simulink model "covering_1_newAxis"  (R2017b)
settings: Solver=VariableStepAuto  StartTime=0.0  StopTime=400  FixedStep=0.0000001  RelTol=1e-3
undefined symbols (not defined in the file): Cwy1, Cwy2, Cx, Jyy, k1_k, k2_k, k2_m, K_thruster, kc, L, lambda11, lambda55, m, Rmin, T_thruster, Vz
libraries: simulink x6, simulink_extras x1
settings Model: PauseTimes=70  NumberOfSteps=10  Creator=Eugene  LastModifiedBy=Eugene
settings DebuggingCC: ParameterOverflowMsg=warning
settings HardwareCC: ProdHWDeviceType=AMD->x86-64 (Windows64)

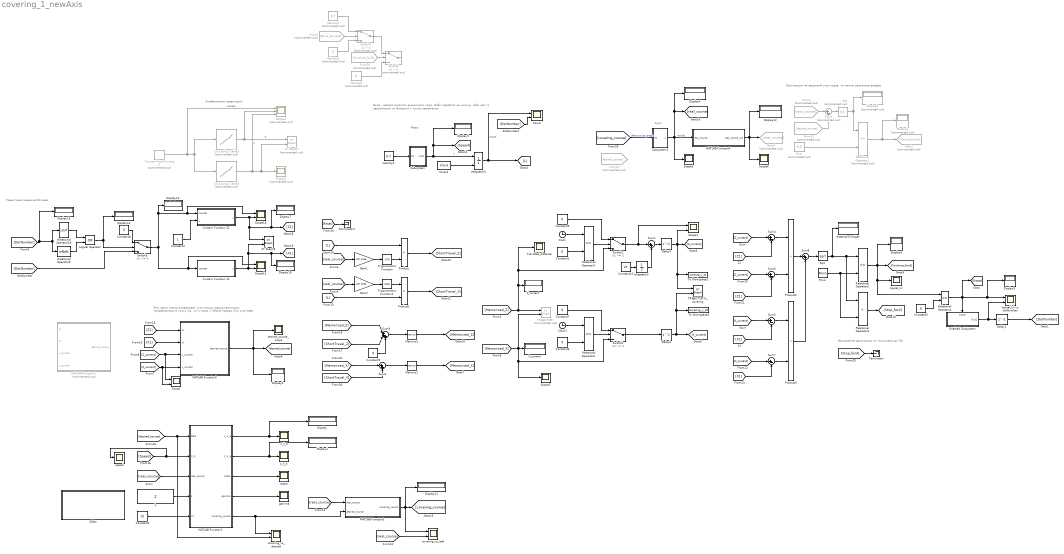
== system covering_1_newAxis ==
  note: Вход - всегда скорость экономного хода. Либо подаётся на контур, либо нет, в зависимости от близости к точке назначения
  note: Марш
  note: angle
  note: Курс
  note: Отображение траектории
  note: Вычисление расстояния от точки-цели до ПА
  note: Если вышли на заданный угол курса, то можно двигаться вперёд
  note: Траектория через switch-case
  note: Эта часть схемы определяет угол между радиус-вектором, направленным в точку (z1, x1) и осью z. Иначе говоря, это угол beta
  1-D Lookup Table2 : Lookup_n-D  Commented=on  NumberOfTableDimensions=1  BreakpointsForDimension1=[0:7]  BreakpointsForDimension1FirstPoint=0  BreakpointsForDimension1DataTypeStr=uint8  Table=[0,0,L,L,2*L,2*L,3*L, 3*L]  TableDataTypeStr=double  InterpMethod=Flat  ExtrapMethod=Cubic spline  RemoveProtectionInput=on  InternalRulePriority=Speed  OutDataTypeStr=double  RndMeth=Zero  InputSameDT=on
  1-D Lookup Table3 : Lookup_n-D  Commented=on  NumberOfTableDimensions=1  BreakpointsForDimension1=[0:7]  BreakpointsForDimension1DataTypeStr=int16  Table=[0,25,25,0,0,25,25,0]  TableDataTypeStr=double  InterpMethod=Flat  RemoveProtectionInput=on  InternalRulePriority=Speed  OutDataTypeStr=double  RndMeth=Zero  InputSameDT=on
  Abs : Abs  Commented=on
  Clock : Clock
  Clock1 : Clock
  Clock2 : simulink_extras/Flip Flops/Clock  period=0.05
  Constant{1,3,5..9} (7 alike) : Constant  Value=0
  Constant10 : Constant  Value=Vz
  Constant2 : Constant  Value=Vz
  Constant4 : Constant  Value=L
  Counter Free-Running2 : simulink/Sources/Counter Free-Running  Commented=on  NumBits=3  tsamp=1
  Custom Function X1 : MATLAB Function  TreatAsAtomicUnit=on
  Custom Function Z1 : MATLAB Function  TreatAsAtomicUnit=on
  Delay1 : Delay  DelayLength=1  SampleTime=0.05
  Delay3 : Delay  DelayLength=1  SampleTime=0.05
  Delay4 : Delay  DelayLength=1  SampleTime=0.05
  Display{,1..2,4..7,9..15} (14 alike) : Display
  Display3 : Display  Commented=on
  Display8 : Display  Commented=on
  Enabled Subsystem : Subsystem  TreatAsAtomicUnit=on
  Error : Constant  Commented=on  Value=0.5
  From11 : From  Commented=on  GotoTag=desired_course
  From2 : From  Commented=on  GotoTag=Move_forward
  From27 : From  Commented=on  GotoTag=desired_course
  From29 : From  Commented=on  GotoTag=Continue_fwrd
  From4 : From  Commented=on  GotoTag=real_course
  Gain1 : Gain  Gain=1/57.2958
  Gain2 : Gain  Gain=1/57.2958
  Goto2 : Goto  Commented=on  GotoTag=Move_forward
  Goto4 : Goto  Commented=on  GotoTag=real_course
  Integrator2 : Integrator
  Integrator3 : Integrator  ExternalReset=rising
  Logical Operator : Logic  Operator=OR  AllPortsSameDT=off  OutDataTypeStr=boolean
  MATLAB Function1 : MATLAB Function  TreatAsAtomicUnit=on
  MATLAB Function2 : MATLAB Function  Commented=on  TreatAsAtomicUnit=on
  MATLAB Function3 : MATLAB Function  TreatAsAtomicUnit=on
  MATLAB Function4 : MATLAB Function  TreatAsAtomicUnit=on
  MATLAB Function5 : MATLAB Function  TreatAsAtomicUnit=on
  Memory1 : Memory
  Memory2 : Memory
  Product{,1..3} (4 alike) : Product
  Relational Operator1 : RelationalOperator  Commented=on  Operator=<=  OutDataTypeStr=boolean  RndMeth=Simplest
  Relational Operator10 : RelationalOperator  Operator=isInf  OutDataTypeStr=boolean  RndMeth=Simplest
  Relational Operator2 : RelationalOperator  OutDataTypeStr=boolean  RndMeth=Simplest
  Relational Operator3 : RelationalOperator  Operator=<  OutDataTypeStr=boolean  RndMeth=Simplest
  Relational Operator4 : RelationalOperator  Operator===  OutDataTypeStr=boolean  RndMeth=Simplest
  Relational Operator5 : RelationalOperator  Operator===  OutDataTypeStr=boolean  RndMeth=Simplest
  Relational Operator6 : RelationalOperator  Operator===  OutDataTypeStr=boolean  RndMeth=Simplest
  Relational Operator9 : RelationalOperator  Operator=isNaN  OutDataTypeStr=boolean  RndMeth=Simplest
  Rmin : Constant  Value=Rmin
  Scope{,1,13..14} (4 alike) : Scope  NumInputPorts=2
  Scope2 : Scope
  Scope3 : Scope  Commented=on  NumInputPorts=3
  Scope4 : Scope  Commented=on
  Scope5 : Scope
  Scope6 : Scope
  Slider : Subsystem  DialogController=hmiCreateDDGDialog  IsWebBlock=on  mask(MWDashboardBlock){webBlockId=306e3f62-3226-42d7-8a36-5c4e99ff92fc, webBlockType=slider, ShowInLibBrowser=on, ShowInitialText=on, HMISrcModelName=covering_1_newAxis}
      mask prompts: webBlockId "WebBlock Id"; webBlockType "WebBlock Type"; HMISrcModelName "Source Model"
      mask help: SimulinkHMI:dialogs:SliderDialogDesc
      mask Help: helpview([docroot '/mapfiles/simulink.map'], 'hmi_slider')
      mask Display:
      | if strcmp(get_param(bdroot(gcb),'BlockDiagramType'), 'library')
      |     image([(matlabroot) '/toolbox/simulink/hmi/icons/Slider.png']);
      | end
  Sqrt : Sqrt  SaturateOnIntegerOverflow=on
  Subsystem : Subsystem
  Subsystem1 : Subsystem
  Sum1 : Sum  Inputs=|++
  Sum2 : Sum  Inputs=|++
  Sum3 : Sum  Commented=on  Inputs=|+-
  Sum{4..7} (4 alike) : Sum  Inputs=|+-
  Sum8 : Sum  Inputs=|++
  Sum9 : Sum  Inputs=|+++
  Switch2 : Switch  Threshold=1
  Switch3 : Switch  Threshold=1
  Switch4 : Switch  Commented=on  Criteria=u2 > Threshold
  Switch5 : Switch  Threshold=1
  Switch6 : Switch  Commented=on  Criteria=u2 > Threshold
  TRAJECTORY : simulink/Sinks/XY Graph  Commented=on  xmin=-1  xmax=10  ymin=-5  ymax=30  st=-1
  TRAJECTORY1_covering : simulink/Sinks/XY Graph  xmin=-1  xmax=10  ymin=-5  ymax=30  st=-1
  Terminator : Terminator
  Terminator1 : Terminator
  To Workspace2 : ToWorkspace  VariableName=covering_z_10  SampleTime=-1
  To Workspace3 : ToWorkspace  VariableName=covering_x_10  SampleTime=-1
  Travelled_distance : Scope
  Trigonometric Function : Trigonometry
  Trigonometric Function1 : Trigonometry  Operator=cos
  Velocity2 : Constant  Value=0.7
  Velocity4 : Constant  Commented=on  Value=0
  Velocity5 : Constant  Commented=on  Value=0.7
  Velocity6 : Constant  Commented=on  Value=0
  XY Graph1 : simulink/Sinks/XY Graph  Commented=on  xmin=-10  xmax=20  ymin=-10  ymax=30  st=-1
  XY Graph5 : simulink/Sinks/XY Graph  xmin=-1  xmax=10  ymin=-5  ymax=30  st=-1
  X_current : Display
  Z_current : Display
  alpha : Scope
  covering_vs_desired : Scope  NumInputPorts=2
  covering_vs_real : Scope  NumInputPorts=2
  desired_course_scope : Scope
  distanceToTarget : Display
  gamma : Scope
  k : Constant  Value=2
  logical_lvl : Scope
  logical_lvl vs dotNumber : Scope  NumInputPorts=2
  "speed " : Scope
  travel : Scope  NumInputPorts=2
  x_V_a : Scope
  z_V_a : Scope
  wires:
  1-D Lookup Table3/1 -> Scope4/1, XY Graph1/2, Scope3/3  "X"
  1-D Lookup Table2/1 -> XY Graph1/1, Scope3/2  "Z"
  Counter Free-Running2/1 -> Scope3/1, 1-D Lookup Table2/1, 1-D Lookup Table3/1  "counter"
  Subsystem/1(Out1) -> [Speed], Display5/1, Integrator3/1  "V"
  [covering_course] -> Subsystem1/1(In1)  "delta course_angle"
  Subsystem1/1(Out1) -> [real_course], Display4/1, Scope5/1, MATLAB Function4/1(real_course)
  Trigonometric Function/1 -> Product/2
  [real_course] -> Gain1/1
  [real_course] -> Gain2/1
  Trigonometric Function1/1 -> Product1/1
  Integrator3/1 -> [L], travel/1  "travel"
  From4/1 -> Sum3/1
  From11/1 -> Sum3/2
  Sum3/1 -> Abs/1
  Error/1 -> Relational Operator1/2
  Relational Operator1/1 -> Goto2/1, Display3/1
  [L] -> Product1/2
  [L] -> Product/1
  Gain1/1 -> Trigonometric Function/1
  Gain2/1 -> Trigonometric Function1/1
  [Z_current] -> Sum4/1
  [Z1] -> Sum4/2
  [X_current] -> Sum5/1
  [X1] -> Sum5/2
  [Z1] -> Sum6/2
  [Z_current] -> Sum6/1
  Sum4/1 -> Product2/1
  Sum6/1 -> Product2/2
  Sum5/1 -> Product3/1
  Sum7/1 -> Product3/2
  [X1] -> Sum7/2
  [X_current] -> Sum7/1
  Product2/1 -> Sum8/1
  Product3/1 -> Sum8/2
  Sum8/1 -> Sqrt/1
  Sqrt/1 -> Relational Operator2/1, Relational Operator3/1, distanceToTarget/1
  Rmin/1 -> Relational Operator2/2, Relational Operator3/2
  Relational Operator3/1 -> [Stop_fwrd]
  Velocity2/1 -> Subsystem/1(In1)
  [Stop_fwrd] -> Terminator/1
  Relational Operator2/1 -> Display6/1, Relational Operator4/1, logical_lvl/1, [Continue_fwrd]
  Constant3/1 -> Relational Operator4/2
  Enabled Subsystem/1(Out1) -> Delay1/1, logical_lvl vs dotNumber/2
  Custom Function X1/1(y) -> Display10/1, [X1], XY Graph5/2, Scope13/2
  Custom Function Z1/1(y) -> Scope14/2, Display7/1, [Z1], XY Graph5/1
  Constant4/1 -> Custom Function Z1/2(L)
  Relational Operator4/1 -> [Reset], Enabled Subsystem/Trigger, logical_lvl vs dotNumber/1, Display9/1
  Switch5/1 -> Display13/1, Scope14/1, Custom Function Z1/1(counter), Scope13/1, Custom Function X1/1(counter)
  Delay1/1 -> [DotNumber]
  Clock2/1 -> Integrator3/2
  [DotNumber] -> travel/2
  Clock/1 -> Relational Operator5/1
  Constant1/1 -> Relational Operator5/2
  Relational Operator5/1 -> Switch2/2
  Constant5/1 -> Switch2/1
  Constant7/1 -> Switch3/1
  Relational Operator6/1 -> Switch3/2
  Constant6/1 -> Relational Operator6/2
  Clock1/1 -> Relational Operator6/1
  [Memorized_X] -> Switch3/3, Scope2/1, TRAJECTORY/2, X_current/1
  Switch3/1 -> Delay3/1
  [DotNumber] -> Switch5/3
  Relational Operator10/1 -> Logical Operator/1
  [DotNumber] -> Display15/1, Relational Operator9/1, Relational Operator10/1
  Relational Operator9/1 -> Logical Operator/2
  Constant8/1 -> Switch5/1
  Logical Operator/1 -> Switch5/2, Display14/1
  Delay3/1 -> [X_current], To Workspace3/1, TRAJECTORY1_covering/2
  Product1/1 -> [ShortTravel_X]
  [Reset] -> Terminator1/1
  Product/1 -> [ShortTravel_Z]
  MATLAB Function5/1(desired_course) -> [desired_course], Display2/1, desired_course_scope/1
  [Z1] -> MATLAB Function5/1(z1)
  [Memorized_X] -> Sum2/1
  Sum2/1 -> Memory1/1
  Memory1/1 -> [Memorized_X]
  [ShortTravel_X] -> Sum2/2
  Abs/1 -> Relational Operator1/1, Display8/1
  [ShortTravel_Z] -> Sum9/2
  Memory2/1 -> [Memorized_Z]
  Sum9/1 -> Memory2/1
  [Memorized_Z] -> Sum9/1
  Constant9/1 -> Sum9/3
  [Memorized_Z] -> Switch2/3, Travelled_distance/1, Z_current/1, TRAJECTORY/1
  Integrator2/1 -> Sum1/2
  Constant10/1 -> Integrator2/1
  Sum1/1 -> Delay4/1
  Switch2/1 -> Sum1/1, Scope1/1
  [desired_course] -> covering_vs_desired/2, MATLAB Function1/1(beta)
  [Speed] -> "speed "/1, MATLAB Function1/2(V_0)
  [real_course] -> MATLAB Function1/3(real_course)
  k/1 -> MATLAB Function1/4(k)
  MATLAB Function1/1(x_V_a) -> Display/1, x_V_a/1
  MATLAB Function1/2(z_V_a) -> Display1/1, z_V_a/1
  MATLAB Function1/3(alpha) -> alpha/1
  MATLAB Function1/4(gamma) -> gamma/1
  [X1] -> MATLAB Function5/2(x1)
  [Z_current] -> MATLAB Function5/3(z_current), Scope/1
  [X_current] -> MATLAB Function5/4(x_current), Scope/2
  MATLAB Function1/5(covering_course) -> MATLAB Function3/2(desired_course), covering_vs_desired/1
  Velocity6/1 -> Switch6/3
  Switch4/1 -> Switch6/1
  From29/1 -> Switch6/2
  From2/1 -> Switch4/2
  Velocity4/1 -> Switch4/3
  Velocity5/1 -> Switch4/1
  MATLAB Function3/1(covering_course) -> covering_vs_real/1, Display11/1, [covering_course]
  [real_course] -> MATLAB Function3/1(real_course)
  MATLAB Function4/1(real_course_out) -> Scope6/1, Goto4/1, Display12/1
  [real_course] -> covering_vs_real/2
  Constant2/1 -> MATLAB Function1/5(Vz)
  Delay4/1 -> To Workspace2/1, TRAJECTORY1_covering/1, [Z_current], Scope1/2

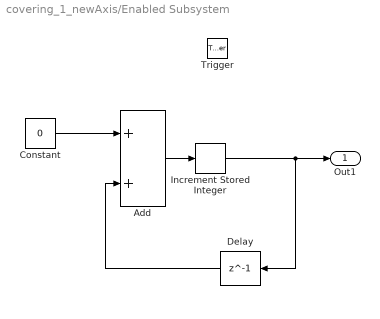
== system covering_1_newAxis/Enabled Subsystem ==
  Trigger : TriggerPort  VariantControl=Variant  PortDimensions=1
  Add : Sum
  Constant : Constant  Value=0
  Delay : Delay  DelayLength=1  InitialCondition=0
  Increment Stored Integer : simulink/Additional Math & Discrete/Additional Math: Increment - Decrement/Increment Stored Integer
      settings: SourceProductName=Simulink
  Out1 : Outport
  wires:
  Constant/1 -> Add/1
  Delay/1 -> Add/2
  Add/1 -> Increment Stored Integer/1
  Increment Stored Integer/1 -> Delay/1, Out1/1

== system covering_1_newAxis/Slider ==

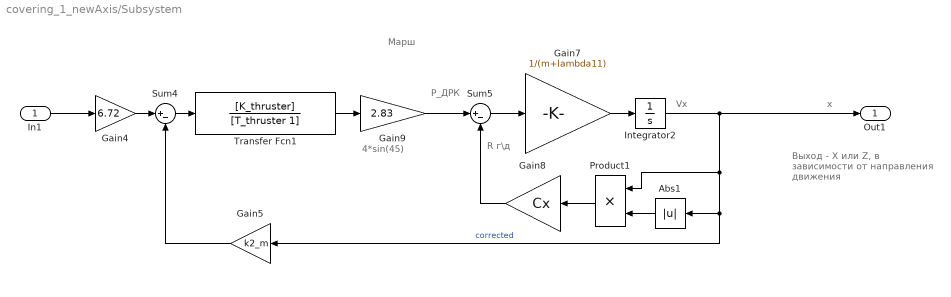
== system covering_1_newAxis/Subsystem ==
  note: Выход - X или Z, в зависимости от направления движения
  note: 4*sin(45)
  note: R г\д
  note: x
  note: Vx
  note: P_ДРК
  note: Марш
  In1 : Inport
  Abs1 : Abs
  Gain4 : Gain  Gain=6.72
  Gain5 : Gain  Gain=k2_m
  Gain7 : Gain  Gain=1/(m+lambda11)
  Gain8 : Gain  Gain=Cx
  Gain9 : Gain  Gain=2.83
  Integrator2 : Integrator  InitialCondition=0.7
  Product1 : Product
  Sum4 : Sum  Inputs=|+-
  Sum5 : Sum  Inputs=|+-
  Transfer Fcn1 : TransferFcn  Numerator=[K_thruster]  Denominator=[T_thruster 1]
  Out1 : Outport
  wires:
  In1/1 -> Gain4/1
  Product1/1 -> Gain8/1
  Gain7/1 -> Integrator2/1
  Gain8/1 -> Sum5/2
  Integrator2/1 -> Out1/1, Gain5/1, Abs1/1, Product1/1  "corrected"
  Transfer Fcn1/1 -> Gain9/1
  Gain4/1 -> Sum4/1
  Sum4/1 -> Transfer Fcn1/1
  Sum5/1 -> Gain7/1
  Gain9/1 -> Sum5/1
  Gain5/1 -> Sum4/2
  Abs1/1 -> Product1/2

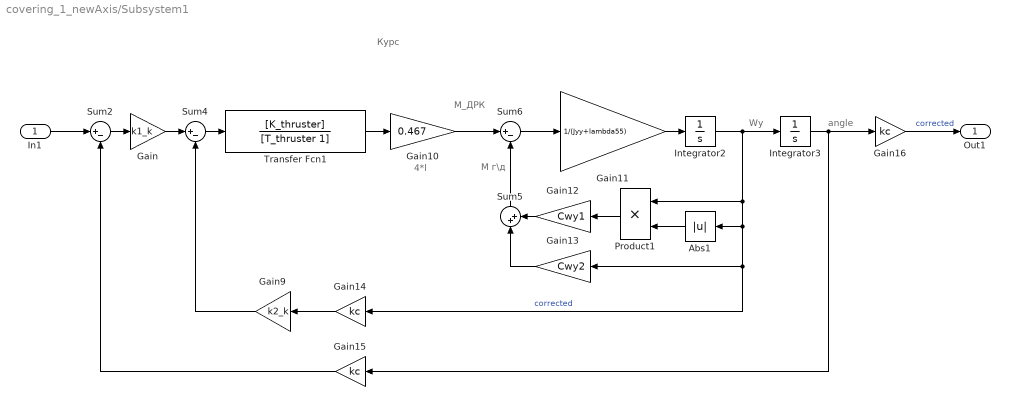
== system covering_1_newAxis/Subsystem1 ==
  note: Курс
  note: Wy
  note: M_ДРК
  note: 4*l
  note: angle
  note: M г\д
  In1 : Inport
  Abs1 : Abs
  Gain : Gain  Gain=k1_k
  Gain10 : Gain  Gain=0.467
  Gain11 : Gain  Gain=1/(Jyy+lambda55)
  Gain12 : Gain  Gain=Cwy1
  Gain13 : Gain  Gain=Cwy2
  Gain14 : Gain  Gain=kc
  Gain15 : Gain  Gain=kc
  Gain16 : Gain  Gain=kc
  Gain9 : Gain  Gain=k2_k
  Integrator2 : Integrator
  Integrator3 : Integrator
  Product1 : Product
  Sum2 : Sum  Inputs=|+-
  Sum4 : Sum  Inputs=|+-
  Sum5 : Sum  Inputs=|++
  Sum6 : Sum  Inputs=|+-
  Transfer Fcn1 : TransferFcn  Numerator=[K_thruster]  Denominator=[T_thruster 1]
  Out1 : Outport
  wires:
  Gain12/1 -> Sum5/2
  Gain10/1 -> Sum6/1
  Product1/1 -> Gain12/1
  Gain11/1 -> Integrator2/1
  Gain9/1 -> Sum4/2
  Gain/1 -> Sum4/1
  Transfer Fcn1/1 -> Gain10/1
  Sum6/1 -> Gain11/1
  Gain14/1 -> Gain9/1
  Gain15/1 -> Sum2/2
  Gain13/1 -> Sum5/1
  Abs1/1 -> Product1/2
  Sum5/1 -> Sum6/2
  Integrator2/1 -> Gain14/1, Gain13/1, Abs1/1, Product1/1, Integrator3/1  "corrected"
  Sum2/1 -> Gain/1
  Integrator3/1 -> Gain16/1, Gain15/1
  Sum4/1 -> Transfer Fcn1/1
  In1/1 -> Sum2/1
  Gain16/1 -> Out1/1  "corrected"

== matlab function covering_1_newAxis/MATLAB Function1 ==
  data: beta input; V_0 input; x_V_a output; z_V_a output; alpha output; gamma output; real_course input; k input; covering_course output; Vz input
function [x_V_a, z_V_a, alpha, gamma, covering_course]  = fcn(beta, V_0, real_course, k, Vz)

% Координаты вектора скорости течения
x_V_current = 0;
z_V_current = Vz;

% Координаты вектора скорости ПА - поменяли
z_V_0 = V_0 * sin(deg2rad(real_course));
x_V_0 = V_0 * cos(deg2rad(real_course));

% Суммарный вектор
x_V_a = x_V_0 + x_V_current;
z_V_a = z_V_0 + z_V_current;

    % Анализ квадранта
    %1
    if (x_V_a >= 0) && (z_V_a >= 0)    
        alpha = rad2deg(atan(z_V_a / x_V_a));
    %2
    elseif (x_V_a >= 0) && (z_V_a < 0)  
        alpha = 360 - rad2deg(atan(abs(z_V_a) / x_V_a));
    %3
    elseif (x_V_a < 0) && (z_V_a < 0)    
        alpha = 180 + rad2deg(atan(abs(z_V_a) / abs(x_V_a)));
    %4
    elseif (x_V_a < 0) && (z_V_a >= 0)    
        alpha = 180 - rad2deg(atan(z_V_a / abs(x_V_a)));   
    else 
        alpha = -1;
    end

% поменяли знак (!)
if (abs(beta - alpha) > 180) && (beta > alpha)
    gamma = (-1) * (360-beta + alpha );
elseif (abs(beta - alpha) > 180) && (beta < alpha)
    gamma = 360-alpha + beta ;
else
    gamma = beta - alpha;
end
%изменено
%if abs(gamma) > 180
%    gamma = (360 - abs(gamma)) * sign(gamma);
%end
%изменено

covering_course = real_course + k * gamma;

while covering_course >= 360
    covering_course =  covering_course - 360;
end

end

== matlab function covering_1_newAxis/MATLAB Function2 ==
  data: z1 input; x1 input; z_current input; desired_course output; x_current input
function desired_course = fcn(z1, x1, z_current, x_current)

if z1 < z_current
    desired_course = 180 - 57.2958*atan((x1-x_current)/(abs(z1-z_current)));
else
    desired_course = 57.2958*atan((x1-x_current)/((z1-z_current)));
end

== matlab function covering_1_newAxis/Custom Function X1 ==
  data: counter input; y output
function y = fcn(counter)

%L = 1.76;

switch counter
    case 1
      y = 25;
    case 2
      y = 0;
    case 3
      y = 0;
    case 4
      y = 25;
    case 5
      y = 25;
    case 6
      y = 0;
    case 7
      y = 0;
    case 8
      y = 25;    
    case 9
      y = 25;
    case 10
      y = 0;
    case 11
      y = 0;    
    case 12
      y = 25;      
   otherwise
      y = 25;
end

== matlab function covering_1_newAxis/Custom Function Z1 ==
  data: counter input; y output; L input
function y = fcn( counter, L)

%L = 1.76;

switch counter
    case 1
      y = L;
    case 2
      y = L;
    case 3
      y = 2*L;
    case 4
      y = 2*L;
    case 5
      y = 3*L;
    case 6
      y = 3*L;
    case 7
      y = 4*L;
    case 8
      y = 4*L;      
    case 9
      y = 5*L; 
    case 10
      y = 5*L;
    case 11
      y = 6*L;
    case 12
      y = 6*L;      
   otherwise
      y = 0;
end

== matlab function covering_1_newAxis/MATLAB Function5 ==
  data: z1 input; x1 input; z_current input; desired_course output; x_current input
function desired_course = fcn(z1, x1, z_current, x_current)

delta_x = x1 - x_current;
delta_z = z1 - z_current;

%1
if (delta_x >= 0) && (delta_z >= 0)
    desired_course = 57.2958*atan(delta_z / delta_x);
%2    
elseif (delta_x >= 0) && (delta_z < 0)
    desired_course = 360 - 57.2958*atan( abs(delta_z) / delta_x);
%3    
elseif (delta_x < 0) && (delta_z < 0)    
    desired_course = 180 + 57.2958*atan(abs(delta_z) / abs(delta_x));
%4    
elseif (delta_x < 0) && (delta_z >= 0)    
    desired_course = 180 - 57.2958*atan( delta_z / abs(delta_x));   
    
else 
    desired_course = -1;
   
end

== matlab function covering_1_newAxis/MATLAB Function3 ==
  data: real_course input; desired_course input; covering_course output
function covering_course   = fcn(real_course, desired_course)

    % предстоит повернуться более чем на 180 градусов
    % текущее положение курса не имеет никакого значения,
    %важно лишь конечное положение.
    % Па должен поворачиват менее чем на 180 градусов
    
    if abs(desired_course - real_course) > 180
        
        if desired_course > 180
            covering_course = desired_course - 360;
        elseif desired_course < -180
            covering_course = 360 + desired_course;
        else
            covering_course = desired_course;
        end
    else
        covering_course = desired_course;
    end
end

== matlab function covering_1_newAxis/MATLAB Function4 ==
  data: real_course input; real_course_out output
function real_course_out   = fcn(real_course)

    % Приводим к стандарту
    if real_course < 0
        real_course_out = 360 - abs(real_course);
    elseif real_course >= 360
        real_course_out = real_course - 360;
    else    
        real_course_out = real_course;
    end

end
